simulink model "SAC"  (R2020b)
settings: Solver=ode4  StartTime=0.0  StopTime=T  FixedStep=s  RelTol=1e-3  EnableMultiTasking=on
values from neighbouring files (symbols this model uses):
  A = [zeros(3,3), eye(3); (-1*(wn)^2)*eye(3),-2*zeta*wn*eye(3)]    [ini_SAC.m]    (also in ini_SACRW.m = [zeros(3,3), eye(3); (-1*(wnn)^2)*eye(3),-2*zetaa*wnn*eye(3))
  a1_B = [1,0,0]'    [ini_SAC.m]    (also in ini_SACRW.m)
  a2_B = [0,1,0]'    [ini_SAC.m]    (also in ini_SACRW.m)
  a3_B = [0,0,1]'    [ini_SAC.m]    (also in ini_SACRW.m)
  alpha = 1    [ini_SAC.m]    (also in ini_SACRW.m)
  B = [zeros(3,3);(wn^2)*eye(3)]    [ini_SAC.m]    (also in ini_SACRW.m = [zeros(3,3);(wnn^2)*eye(3)])
  C = [eye(6)]    [ini_SAC.m]    (also in ini_SACRW.m)
  D = [zeros(6,3)]    [ini_SAC.m]    (also in ini_SACRW.m)
  gIE = 1e5*(eye(3))    [ini_SAC.m]    (also in ini_SACRW.m = 1e3*(eye(3)))
  gIU = 1e3*(eye(3))    [ini_SAC.m]    (also in ini_SACRW.m)
  gIX = 1e3*(eye(6))    [ini_SAC.m]    (also in ini_SACRW.m)
  gPE = 1e5*(eye(3))    [ini_SAC.m]    (also in ini_SACRW.m = 1e3*(eye(3)))
  gPU = 1e3*(eye(3))    [ini_SAC.m]    (also in ini_SACRW.m)
  gPX = 1e3*(eye(6))    [ini_SAC.m]    (also in ini_SACRW.m)
  ha1_B_ini = ha1_ini*a1_B    [ini_SAC.m]    (also in ini_SACRW.m)
  ha2_B_ini = ha2_ini*a2_B    [ini_SAC.m]    (also in ini_SACRW.m)
  ha3_B_ini = ha3_ini*a3_B    [ini_SAC.m]    (also in ini_SACRW.m)
  Jsc = [114 0 0;0 86 0;0 0 87]    [ini_SAC.m]    (also in ini_SACRW.m = 1*[114 0 0;0 86 0;0 0 87])
  q_d = [0 0 0 1]'    [ini_SAC.m]    (also in ini_SACRW.m)
  r_I_ini = [-0.1 0.5 1.0]    [ini_SAC.m]
  rw_t = 0.01    [ini_SAC.m]    (also in ini_SACRW.m)
undefined symbols (not defined in the file or in its folder): gammaE, gammaU, gammaX
libraries: simulink_extras x3
settings Model: Creator=hoomanrajaee  LastModifiedBy=Graham Stokes
settings DataIOCC: LimitDataPoints=on  SaveFormat=Array  SignalLoggingSaveFormat=ModelDataLogs  ReturnWorkspaceOutputs=off
settings OptimizationCC: LifeSpan=inf
settings DebuggingCC: UnderspecifiedInitializationDetection=Classic  MergeDetectMultiDrivingBlocksExec=none  SolverPrmCheckMsg=warning  MultiTaskDSMMsg=warning  MultiTaskCondExecSysMsg=none  AllowSymbolicDim=off  StateNameClashWarn=warning  SFUnexpectedBacktrackingDiag=warning  SFNoUnconditionalDefaultTransitionDiag=warning  UnderSpecifiedDimensionMsg=warning  ArithmeticOperatorsInVariantConditions=warning
settings HardwareCC: ProdBitPerPointer=32  ProdBitPerSizeT=32  ProdBitPerPtrDiffT=32  ProdLargestAtomicFloat=None  ProdIntDivRoundTo=Undefined  ProdEndianess=Unspecified  ProdWordSize=32  ProdHWDeviceType=32-bit Generic
settings ModelReferenceCC: PropagateSignalLabelsOutOfModel=off
settings SFSimCC: SimUseLocalCustomCode=off  CustomCodeUndefinedFunction=UseInterfaceOnly
settings RTWCC: RTWUseLocalCustomCode=off
settings CodeAppCC: StateflowObjectComments=on
settings GRTTargetCC: TargetLangStandard=C89/C90 (ANSI)
settings ConfigComp: CovMetricSettings=dw  CovSaveCumulativeToWorkspaceVar=on  CovSaveSingleToWorkspaceVar=on  CovExternalEMLEnable=off

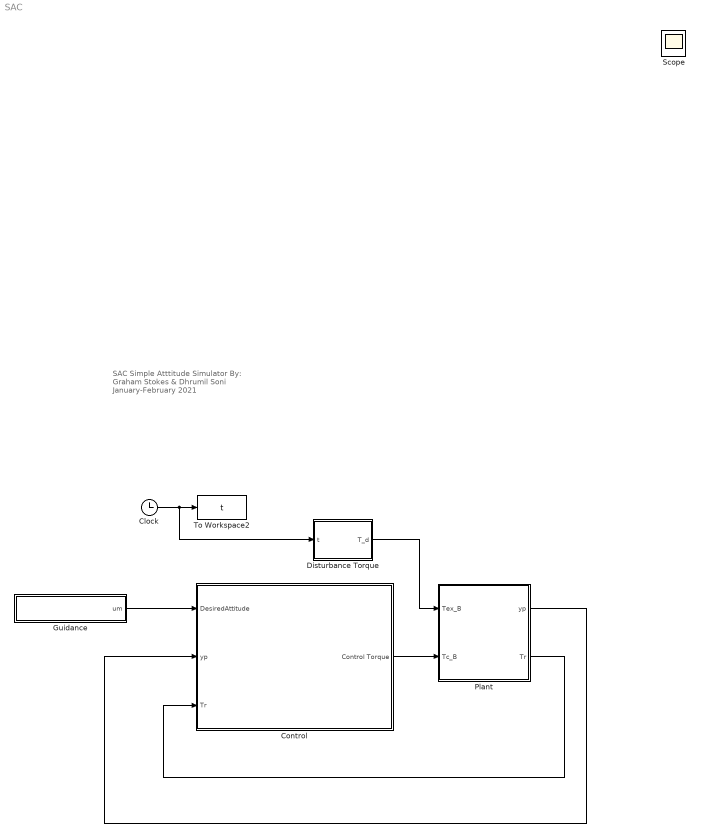
== system SAC ==
  note: SAC Simple Atttitude Simulator
      | By: Graham Stokes & Dhrumil Soni
      | January-February 2021
  Clock : Clock
  Control : Subsystem
  Disturbance Torque : MATLAB Function  TreatAsAtomicUnit=on
  "Guidance " : Subsystem
  Plant : Subsystem
  To Workspace2 : ToWorkspace  VariableName=t  SampleTime=-1
  Scope : Scope
  wires:
  Clock/1 -> Disturbance Torque/1(t), To Workspace2/1
  "Guidance "/1(um) -> Control/1(DesiredAttitude)
  Control/1(Control Torque) -> Plant/2(Tc_B)
  Plant/1("yp ") -> Control/2(yp)
  Plant/2("Tr ") -> Control/3(Tr)
  Disturbance Torque/1(T_d) -> Plant/1(Tex_B)

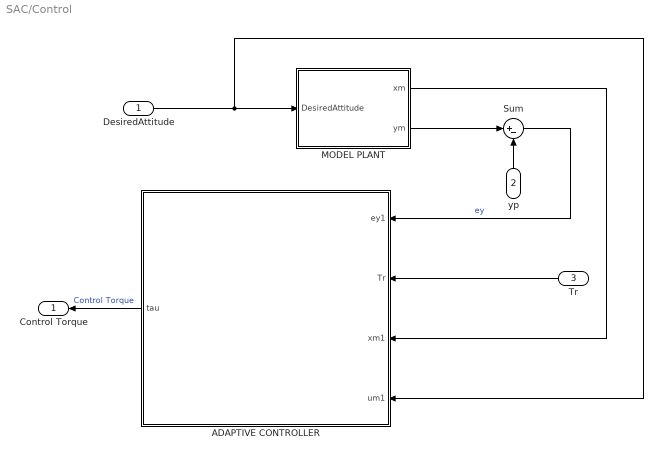
== system SAC/Control ==
  DesiredAttitude : Inport
  yp : Inport  Port=2
  Tr : Inport  Port=3
  ADAPTIVE CONTROLLER : Subsystem
      settings: AttributesFormatString=Adaptive Controller
  MODEL PLANT : Subsystem
  Sum : Sum  Inputs=|+-
  Control Torque : Outport
  wires:
  DesiredAttitude/1 -> ADAPTIVE CONTROLLER/4(um1), MODEL PLANT/1(DesiredAttitude)
  MODEL PLANT/2(ym) -> Sum/1
  Tr/1 -> ADAPTIVE CONTROLLER/2(Tr)
  ADAPTIVE CONTROLLER/1(tau) -> Control Torque/1  "Control Torque"
  yp/1 -> Sum/2
  Sum/1 -> ADAPTIVE CONTROLLER/1(ey1)  "ey"
  MODEL PLANT/1(xm) -> ADAPTIVE CONTROLLER/3(xm1)

== system SAC/Guidance  ==
  MRP : MATLAB Function  TreatAsAtomicUnit=on
  To Workspace : ToWorkspace  VariableName=um  SaveFormat=Timeseries  SampleTime=-1
  q_d1 : Constant  Value=q_d
  um : Outport
  wires:
  MRP/1(r) -> To Workspace/1, um/1  "um"
  q_d1/1 -> MRP/1(qsc_I_sign)

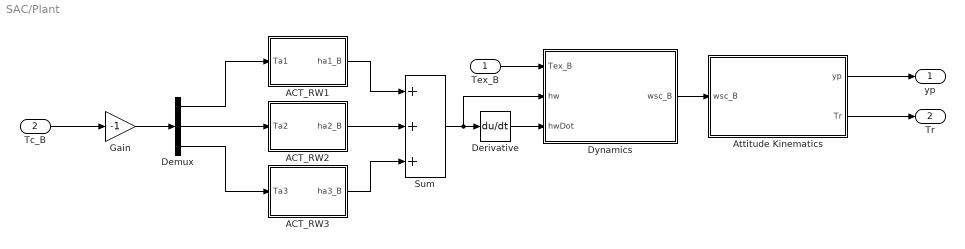
== system SAC/Plant ==
  Tex_B : Inport
  Tc_B : Inport  Port=2
  ACT_RW1 : Subsystem
  ACT_RW2 : Subsystem
  ACT_RW3 : Subsystem
  Attitude Kinematics : Subsystem
  Demux : Demux  Outputs=3
  Derivative : Derivative
  Dynamics : Subsystem
  Gain : Gain  Gain=-1
  Sum : Sum  Inputs=+++
  "yp " : Outport
  "Tr " : Outport  Port=2
  wires:
  Attitude Kinematics/2(Tr) -> "Tr "/1
  Attitude Kinematics/1(yp) -> "yp "/1
  Demux/3 -> ACT_RW3/1(Ta3)
  ACT_RW2/1(ha2_B) -> Sum/2
  Demux/1 -> ACT_RW1/1(Ta1)
  ACT_RW1/1(ha1_B) -> Sum/1
  ACT_RW3/1(ha3_B) -> Sum/3
  Sum/1 -> Derivative/1, Dynamics/2(hw)
  Demux/2 -> ACT_RW2/1(Ta2)
  Derivative/1 -> Dynamics/3(hwDot)
  Tex_B/1 -> Dynamics/1(Tex_B)
  Tc_B/1 -> Gain/1
  Dynamics/1(wsc_B) -> Attitude Kinematics/1(wsc_B)
  Gain/1 -> Demux/1

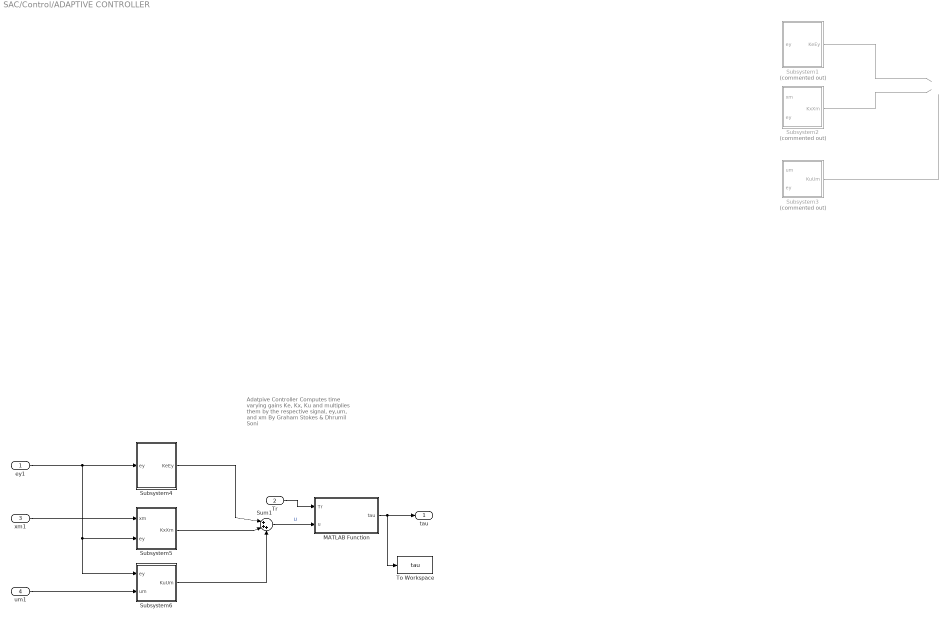
== system SAC/Control/ADAPTIVE CONTROLLER ==
  note: Adatpive Controller
      | Computes time varying gains Ke, Kx, Ku and multiplies them by the respective signal, ey,um, and xm
      | By Graham Stokes & Dhrumil Soni
  ey1 : Inport
  Tr : Inport  Port=2
  xm1 : Inport  Port=3
  um1 : Inport  Port=4
  MATLAB Function : MATLAB Function  TreatAsAtomicUnit=on
  Subsystem1 : Subsystem  Commented=on
  Subsystem2 : Subsystem  Commented=on
  Subsystem3 : Subsystem  Commented=on
  Subsystem4 : Subsystem
  Subsystem5 : Subsystem
  Subsystem6 : Subsystem
  Sum1 : Sum  Inputs=|+++
  To Workspace : ToWorkspace  VariableName=tau  SaveFormat=Timeseries  SampleTime=-1
  tau : Outport
  wires:
  Tr/1 -> MATLAB Function/1(Tr)
  Sum1/1 -> MATLAB Function/2(u)  "U"
  MATLAB Function/1(tau) -> tau/1, To Workspace/1
  Subsystem5/1(KxXm) -> Sum1/2
  Subsystem4/1(KeEy) -> Sum1/1
  Subsystem6/1(KuUm) -> Sum1/3
  um1/1 -> Subsystem6/2(um)
  xm1/1 -> Subsystem5/1(xm)
  ey1/1 -> Subsystem4/1(ey), Subsystem6/1(ey), Subsystem5/2(ey)
  Subsystem2/1(KxXm) -> ?
  Subsystem3/1(KuUm) -> ?
  Subsystem1/1(KeEy) -> ?

== system SAC/Control/MODEL PLANT ==
  note: Model Plant
      |
      | State space model outputing the desired response. Parse Y outputs the damped position respoonse of the model.
      |
      | By Graham Stokes & Dhrumil Soni
  DesiredAttitude : Inport
  Constant : Constant  Value=alpha
  MATLAB Function : MATLAB Function  TreatAsAtomicUnit=on
  State-Space Model : StateSpace  A=A  B=B  C=C  D=D  InitialCondition=[r_I_ini(1);r_I_ini(2);r_I_ini(3);0;0;0]
  xm : Outport
  ym : Outport  Port=2
  wires:
  DesiredAttitude/1 -> State-Space Model/1
  MATLAB Function/1(ym) -> ym/1
  Constant/1 -> MATLAB Function/2(alpha)
  State-Space Model/1 -> MATLAB Function/1(X), xm/1

== system SAC/Plant/ACT_RW1 ==
  note: First order transfer function from actuated torque to control torque. By M.Sidi
  Ta1 : Inport
  Constant1 : Constant  Value=a1_B
  Integrator : Integrator  InitialCondition=ha1_B_ini
  Product1 : Product
  Transfer Fcn (with initial states) : simulink_extras/Additional Linear/Transfer Fcn (with initial states)  N=[1]  D=[rw_t 1]  X0=.5
  ha1_B : Outport
  wires:
  Product1/1 -> ha1_B/1
  Integrator/1 -> Product1/1
  Constant1/1 -> Product1/2
  Ta1/1 -> Transfer Fcn (with initial states)/1
  Transfer Fcn (with initial states)/1 -> Integrator/1  "Tc1"

== system SAC/Plant/ACT_RW2 ==
  Ta2 : Inport
  Constant1 : Constant  Value=a2_B
  Integrator : Integrator  InitialCondition=ha2_B_ini
  Product1 : Product
  Transfer Fcn (with initial states) : simulink_extras/Additional Linear/Transfer Fcn (with initial states)  N=[1]  D="[rw_t  1]"  X0=.5
  ha2_B : Outport
  wires:
  Constant1/1 -> Product1/2
  Product1/1 -> ha2_B/1
  Integrator/1 -> Product1/1
  Ta2/1 -> Transfer Fcn (with initial states)/1
  Transfer Fcn (with initial states)/1 -> Integrator/1  "Tc1"

== system SAC/Plant/ACT_RW3 ==
  Ta3 : Inport
  Constant1 : Constant  Value=a3_B
  Integrator : Integrator  InitialCondition=ha3_B_ini
  Product1 : Product
  Transfer Fcn (with initial states) : simulink_extras/Additional Linear/Transfer Fcn (with initial states)  N=[1]  D="[rw_t  1]"  X0=.5
  ha3_B : Outport
  wires:
  Constant1/1 -> Product1/2
  Product1/1 -> ha3_B/1
  Integrator/1 -> Product1/1
  Ta3/1 -> Transfer Fcn (with initial states)/1
  Transfer Fcn (with initial states)/1 -> Integrator/1  "Tc3"

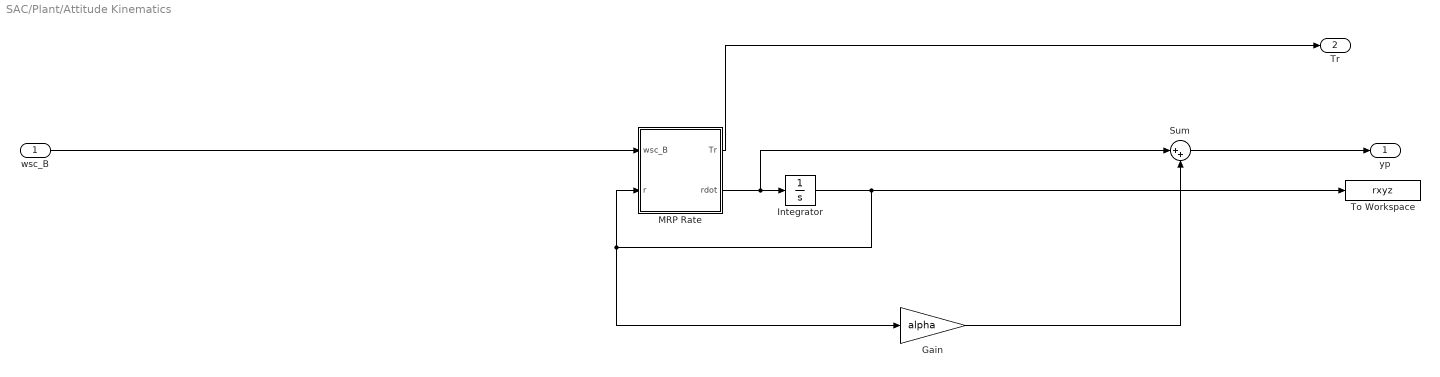
== system SAC/Plant/Attitude Kinematics ==
  wsc_B : Inport
  Gain : Gain  Gain=alpha
  Integrator : Integrator  InitialCondition=r_I_ini
  MRP Rate : MATLAB Function  TreatAsAtomicUnit=on
  Sum : Sum  Inputs=|++
  To Workspace : ToWorkspace  VariableName=rxyz  SaveFormat=Timeseries  SampleTime=-1
  yp : Outport
  Tr : Outport  Port=2
  wires:
  MRP Rate/2(rdot) -> Sum/1, Integrator/1
  Sum/1 -> yp/1
  Gain/1 -> Sum/2
  MRP Rate/1(Tr) -> Tr/1
  wsc_B/1 -> MRP Rate/1(wsc_B)
  Integrator/1 -> Gain/1, MRP Rate/2(r), To Workspace/1

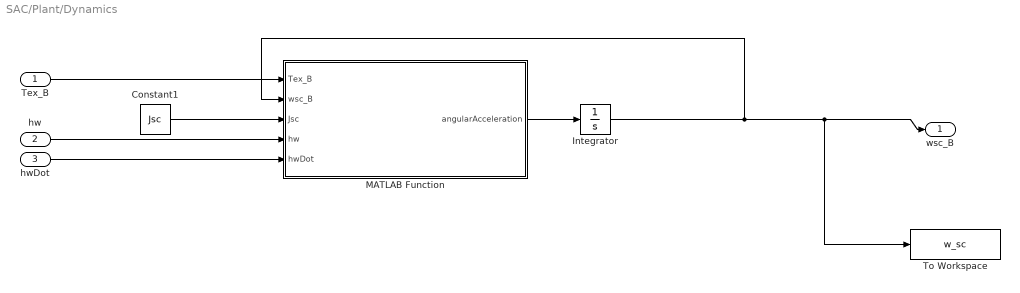
== system SAC/Plant/Dynamics ==
  Tex_B : Inport
  hw : Inport  Port=2
  hwDot : Inport  Port=3
  Constant1 : Constant  Value=Jsc
  Integrator : Integrator  InitialCondition=[0 0 0]';
  MATLAB Function : MATLAB Function  TreatAsAtomicUnit=on
  To Workspace : ToWorkspace  VariableName=w_sc  SaveFormat=Timeseries  SampleTime=-1
  wsc_B : Outport
  wires:
  Integrator/1 -> MATLAB Function/2(wsc_B), To Workspace/1, wsc_B/1
  Constant1/1 -> MATLAB Function/3(Jsc)
  MATLAB Function/1(angularAcceleration) -> Integrator/1
  Tex_B/1 -> MATLAB Function/1(Tex_B)
  hw/1 -> MATLAB Function/4(hw)
  hwDot/1 -> MATLAB Function/5(hwDot)

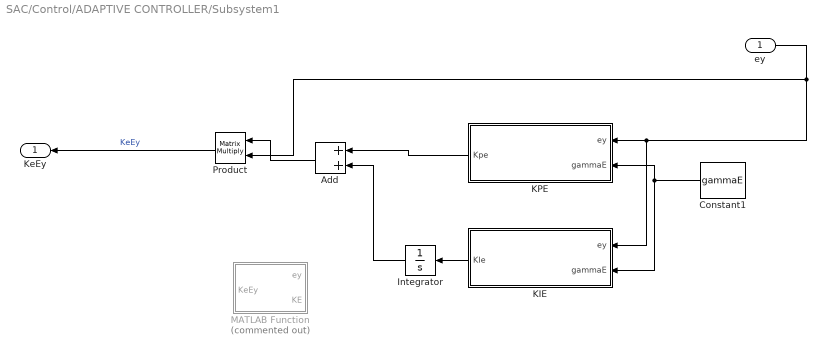
== system SAC/Control/ADAPTIVE CONTROLLER/Subsystem1 ==
  ey : Inport
  Add : Sum
  Constant1 : Constant  Value=gammaE
  Integrator : Integrator
  KIE : MATLAB Function  TreatAsAtomicUnit=on
  KPE : MATLAB Function  TreatAsAtomicUnit=on
  MATLAB Function : MATLAB Function  Commented=on  TreatAsAtomicUnit=on
  Product : Product  Multiplication=Matrix(*)
  KeEy : Outport
  wires:
  ey/1 -> Product/2, KPE/1(ey), KIE/1(ey)
  KPE/1(Kpe) -> Add/1
  KIE/1(KIe) -> Integrator/1
  Constant1/1 -> KPE/2(gammaE), KIE/2(gammaE)
  Product/1 -> KeEy/1  "KeEy"
  Integrator/1 -> Add/2
  Add/1 -> Product/1

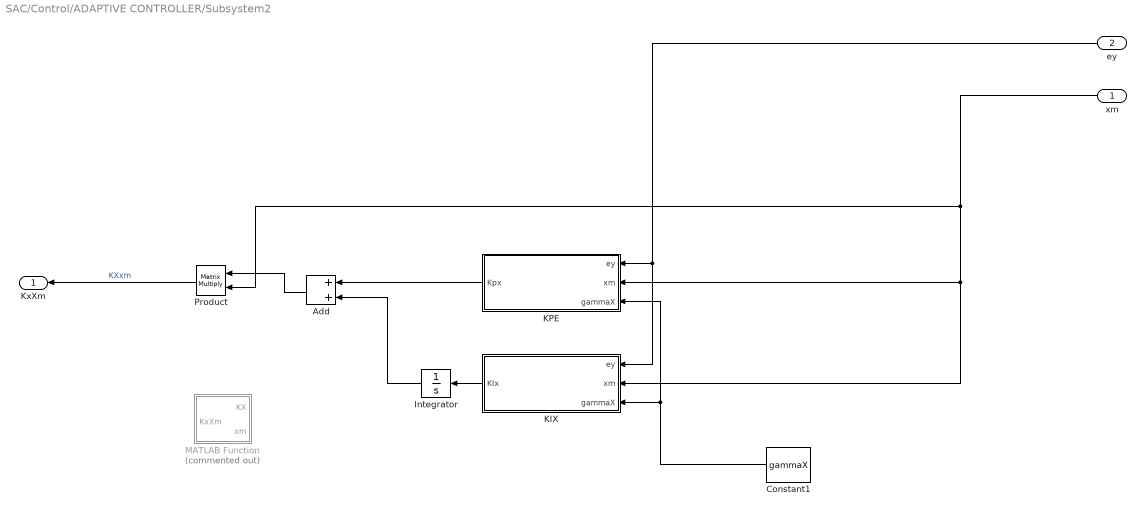
== system SAC/Control/ADAPTIVE CONTROLLER/Subsystem2 ==
  xm : Inport
  ey : Inport  Port=2
  Add : Sum
  Constant1 : Constant  Value=gammaX
  Integrator : Integrator
  KIX : MATLAB Function  TreatAsAtomicUnit=on
  KPE : MATLAB Function  TreatAsAtomicUnit=on
  MATLAB Function : MATLAB Function  Commented=on  TreatAsAtomicUnit=on
  Product : Product  Multiplication=Matrix(*)
  KxXm : Outport
  wires:
  ey/1 -> KPE/1(ey), KIX/1(ey)
  xm/1 -> Product/2, KIX/2(xm), KPE/2(xm)
  Add/1 -> Product/1
  Integrator/1 -> Add/2
  KPE/1(Kpx) -> Add/1
  Constant1/1 -> KPE/3(gammaX), KIX/3(gammaX)
  Product/1 -> KxXm/1  "KXxm"
  KIX/1(KIx) -> Integrator/1

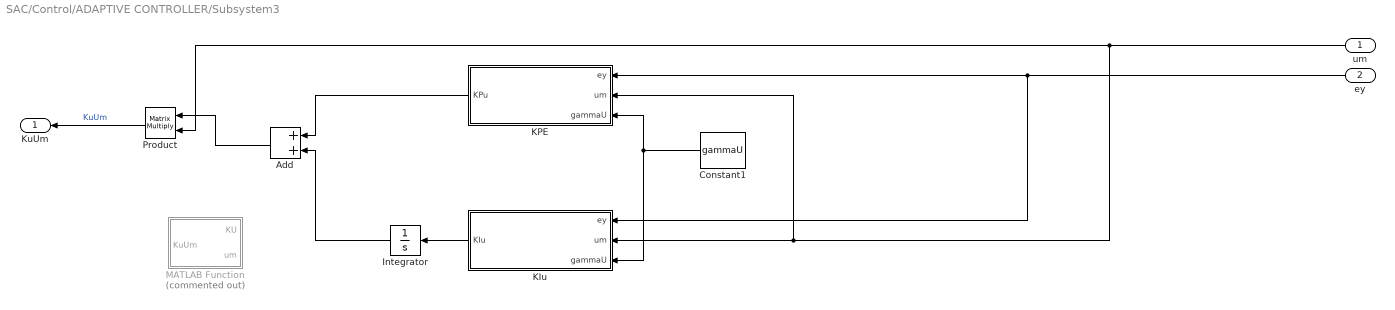
== system SAC/Control/ADAPTIVE CONTROLLER/Subsystem3 ==
  um : Inport
  ey : Inport  Port=2
  Add : Sum
  Constant1 : Constant  Value=gammaU
  Integrator : Integrator
  KIu : MATLAB Function  TreatAsAtomicUnit=on
  KPE : MATLAB Function  TreatAsAtomicUnit=on
  MATLAB Function : MATLAB Function  Commented=on  TreatAsAtomicUnit=on
  Product : Product  Multiplication=Matrix(*)
  KuUm : Outport
  wires:
  Product/1 -> KuUm/1  "KuUm"
  KIu/1(KIu) -> Integrator/1
  ey/1 -> KPE/1(ey), KIu/1(ey)
  KPE/1(KPu) -> Add/1
  Integrator/1 -> Add/2
  Constant1/1 -> KIu/3(gammaU), KPE/3(gammaU)
  um/1 -> Product/2, KPE/2(um), KIu/2(um)
  Add/1 -> Product/1

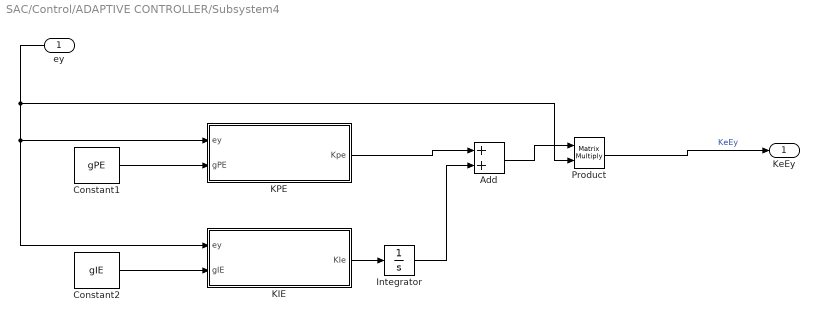
== system SAC/Control/ADAPTIVE CONTROLLER/Subsystem4 ==
  ey : Inport
  Add : Sum
  Constant1 : Constant  Value=gPE
  Constant2 : Constant  Value=gIE
  Integrator : Integrator
  KIE : MATLAB Function  TreatAsAtomicUnit=on
  KPE : MATLAB Function  TreatAsAtomicUnit=on
  Product : Product  Multiplication=Matrix(*)
  KeEy : Outport
  wires:
  ey/1 -> KPE/1(ey), KIE/1(ey), Product/2
  KPE/1(Kpe) -> Add/1
  KIE/1(KIe) -> Integrator/1
  Constant1/1 -> KPE/2(gPE)
  Product/1 -> KeEy/1  "KeEy"
  Integrator/1 -> Add/2
  Add/1 -> Product/1
  Constant2/1 -> KIE/2(gIE)

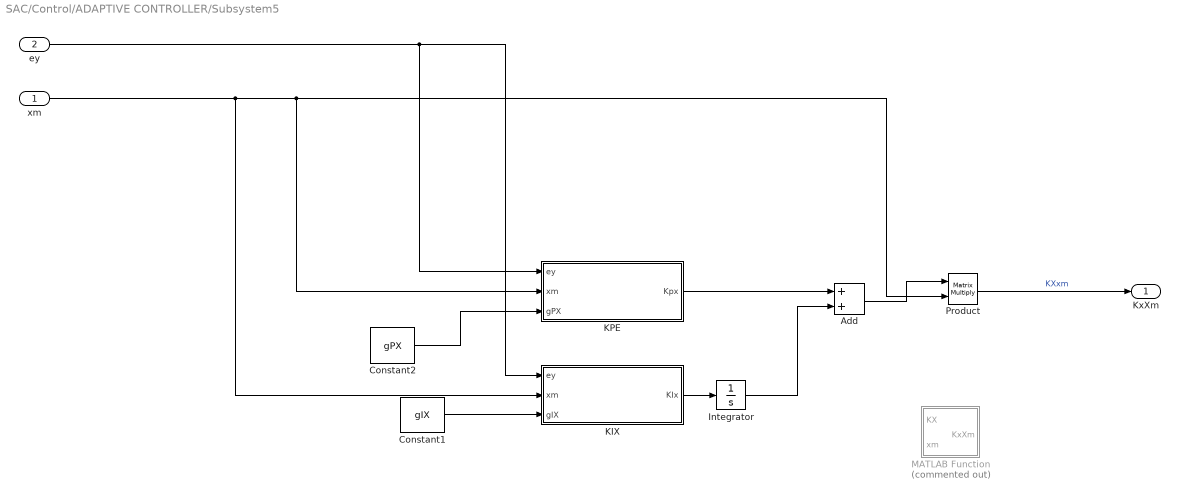
== system SAC/Control/ADAPTIVE CONTROLLER/Subsystem5 ==
  xm : Inport
  ey : Inport  Port=2
  Add : Sum
  Constant1 : Constant  Value=gIX
  Constant2 : Constant  Value=gPX
  Integrator : Integrator
  KIX : MATLAB Function  TreatAsAtomicUnit=on
  KPE : MATLAB Function  TreatAsAtomicUnit=on
  MATLAB Function : MATLAB Function  Commented=on  TreatAsAtomicUnit=on
  Product : Product  Multiplication=Matrix(*)
  KxXm : Outport
  wires:
  ey/1 -> KPE/1(ey), KIX/1(ey)
  xm/1 -> KPE/2(xm), Product/2, KIX/2(xm)
  Add/1 -> Product/1
  Integrator/1 -> Add/2
  KPE/1(Kpx) -> Add/1
  Constant1/1 -> KIX/3(gIX)
  Product/1 -> KxXm/1  "KXxm"
  KIX/1(KIx) -> Integrator/1
  Constant2/1 -> KPE/3(gPX)

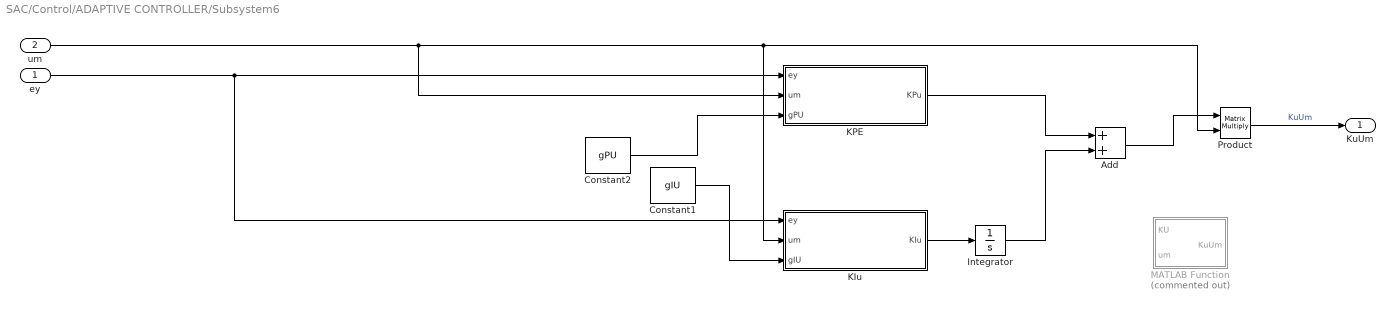
== system SAC/Control/ADAPTIVE CONTROLLER/Subsystem6 ==
  ey : Inport
  um : Inport  Port=2
  Add : Sum
  Constant1 : Constant  Value=gIU
  Constant2 : Constant  Value=gPU
  Integrator : Integrator
  KIu : MATLAB Function  TreatAsAtomicUnit=on
  KPE : MATLAB Function  TreatAsAtomicUnit=on
  MATLAB Function : MATLAB Function  Commented=on  TreatAsAtomicUnit=on
  Product : Product  Multiplication=Matrix(*)
  KuUm : Outport
  wires:
  Product/1 -> KuUm/1  "KuUm"
  KIu/1(KIu) -> Integrator/1
  ey/1 -> KPE/1(ey), KIu/1(ey)
  KPE/1(KPu) -> Add/1
  Integrator/1 -> Add/2
  Constant1/1 -> KIu/3(gIU)
  um/1 -> KIu/2(um), Product/2, KPE/2(um)
  Add/1 -> Product/1
  Constant2/1 -> KPE/3(gPU)

== matlab function SAC/Plant/Attitude Kinematics/MRP Rate ==
  data: Tr output; wsc_B input; r input; rdot output
function [Tr,rdot]= fcn(wsc_B,r)
        
    Tr = zeros(3,3); 
    Tr = 0.25*((1-transpose(r)*r)*eye(3)+2*skew(r)+2*r*transpose(r));
   
    TrInv = zeros(3,3); 
    TrInv = 4*(((1+transpose(r)*r)^-2)*(1-transpose(r)*r)*eye(3)-2*skew(r)+2*r*transpose(r));
    
    %set size of T(r) matrix 
    rdot = Tr*wsc_B; 
    
end

== matlab function SAC/Plant/Dynamics/MATLAB Function ==
  data: Tex_B input; angularAcceleration output; wsc_B input; Jsc input; hw input; hwDot input
function angularAcceleration = EulerDynamics(Tex_B,wsc_B,Jsc,hw,hwDot)
%% Euler's Equation of Motion
%Graham Stokes
%hw is the reaction wheel angular momentum

J_b = Jsc;              %inertia of s/c (3x1)
%wsc_B                  %ang vel of s/c (3x1)
T = Tex_B;              %torque from pert. model (3x1)
wsc_skew = skew(wsc_B); %skew matrix (3x3)

angularAcceleration = inv(J_b)*(T-(wsc_skew*(J_b*wsc_B + hw))- hwDot); %(3x1)


end

== matlab function SAC/Disturbance Torque ==
  data: t input; T_d output
function T_d = Dist(t)
%Perturbation model by Dr.Ulrich

%Written by Graham Stokes 

% Approximates magnetic torques, atm. drag, solar pressures, and 
% gravity gradients based by a first order fourier series 

%mu = grav. parameter 
%a = radius of orbit 
%n = orbital mean motion 
%a0,a1,b1 represent the coefficients 
%Td = pert torques



    mu = 398600.4418;
    RE = 6378.137; 
    a = RE + 728;       
    n = sqrt(mu/a^3); 
    a0 = 10^-6*[-4.14 10.2 -5.07]';
    a1 = 10^-6.*[6.92 -9.05 3.40]';
    b1 = 10^-6.*[-8.77 1.33 7.56]'; 

    T_d = a0 + a1*cos(n*t) + b1*sin(n*t); 

end

== matlab function SAC/Guidance /MRP ==
  data: qsc_I_sign input; r output
function r  = QuatToMRP(qsc_I_sign)

%Graham Stokes 
%converts quaternion (4x1) to MRP (3x1)

    q = qsc_I_sign; 
    r = zeros(3,1); 
    eps = zeros(3,1); 
    
    eps(1) = q(1);
    eps(2) = q(2); 
    eps(3) = q(3); 
    
    r = eps/(1+q(4)); 
    
end

== matlab function SAC/Control/ADAPTIVE CONTROLLER/Subsystem1/KIE ==
  data: ey input; KIe output; gammaE input
function KIe = KIE(ey,gammaE)
    KIe = ey*(ey')*gammaE;
end

== matlab function SAC/Control/ADAPTIVE CONTROLLER/Subsystem4/KIE ==
  data: ey input; KIe output; gIE input
function KIe = KIE(ey,gIE)
    KIe = ey*(ey')*gIE;
end

== matlab function SAC/Control/ADAPTIVE CONTROLLER/Subsystem4/KPE ==
  data: ey input; Kpe output; gPE input
function Kpe = KPE(ey,gPE)
    Kpe = ey*(ey')*gPE;
end

== matlab function SAC/Control/ADAPTIVE CONTROLLER/Subsystem5/KIX ==
  data: ey input; KIx output; xm input; gIX input
function KIx = KIX(ey, xm,gIX)
    KIx = (ey)*(xm')*gIX;
end

== matlab function SAC/Control/ADAPTIVE CONTROLLER/Subsystem5/KPE ==
  data: ey input; Kpx output; xm input; gPX input
function Kpx = KPX(ey, xm,gPX)
    Kpx = (ey)*(xm')*gPX;
end

== matlab function SAC/Control/ADAPTIVE CONTROLLER/Subsystem5/MATLAB Function ==
  data: KX input; xm input; KxXm output
function  KxXm = KX(KX, xm)

KxXm = KX*xm

end

== matlab function SAC/Control/ADAPTIVE CONTROLLER/Subsystem6/KIu ==
  data: ey input; um input; KIu output; gIU input
function KIu = KIU(ey,um,gIU)
    KIu = ey*(um')*gIU;
end

== matlab function SAC/Control/ADAPTIVE CONTROLLER/Subsystem6/KPE ==
  data: ey input; KPu output; um input; gPU input
function KPu = KPU(ey,um,gPU)
    KPu = ey*(um')*gPU;
end

== matlab function SAC/Control/ADAPTIVE CONTROLLER/Subsystem6/MATLAB Function ==
  data: KU input; um input; KuUm output
function  KuUm = fcn(KU, um)

KuUm = KU*um

end

== matlab function SAC/Control/ADAPTIVE CONTROLLER/Subsystem1/KPE ==
  data: ey input; Kpe output; gammaE input
function Kpe = KPE(ey,gammaE)
    Kpe = ey*(ey')*gammaE;
end

== matlab function SAC/Control/ADAPTIVE CONTROLLER/Subsystem2/KIX ==
  data: ey input; KIx output; xm input; gammaX input
function KIx = KIX(ey, xm,gammaX)
    KIx = (ey)*(xm')*gammaX;
end

== matlab function SAC/Control/ADAPTIVE CONTROLLER/Subsystem2/KPE ==
  data: ey input; Kpx output; xm input; gammaX input
function Kpx = KPX(ey, xm,gammaX)
    Kpx = (ey)*(xm')*gammaX;
end

== matlab function SAC/Control/ADAPTIVE CONTROLLER/Subsystem3/KIu ==
  data: ey input; um input; KIu output; gammaU input
function KIu = KIU(ey,um,gammaU)
    KIu = ey*(um')*gammaU;
end

== matlab function SAC/Control/ADAPTIVE CONTROLLER/Subsystem3/KPE ==
  data: ey input; KPu output; um input; gammaU input
function KPu = KPU(ey,um,gammaU)
    KPu = ey*(um')*gammaU;
end

== matlab function SAC/Control/ADAPTIVE CONTROLLER/MATLAB Function ==
  data: Tr input; u input; tau output
function tau = torqueGen(Tr, u )
%Compute torque signal
tau = Tr'*u;

end

== matlab function SAC/Control/ADAPTIVE CONTROLLER/Subsystem1/MATLAB Function ==
  data: ey input; KE input; KeEy output
function KeEy = fcn(ey,KE)

KeEy = KE*ey

end

== matlab function SAC/Control/MODEL PLANT/MATLAB Function ==
  data: X input; ym output; alpha input
function ym = parseY(X, alpha)
    % Graham Stokes
    %X = (6x1)state vector 
    %ym = (3x1)state output
        %Includes position and damping value--> similar to plant output
        
    ym = alpha*eye(3)*X(1:3) + X(4:6);
    
end

== matlab function SAC/Control/ADAPTIVE CONTROLLER/Subsystem3/MATLAB Function ==
  data: KU input; um input; KuUm output
function  KuUm = fcn(KU, um)

KuUm = KU*um

end

== matlab function SAC/Control/ADAPTIVE CONTROLLER/Subsystem2/MATLAB Function ==
  data: KX input; xm input; KxXm output
function  KxXm = KX(KX, xm)

KxXm = KX*xm

end
